simulink model "project2_animation"  (R2017a)
settings: Solver=FixedStepDiscrete  StartTime=0.0  StopTime=1000.0  FixedStep=0.1  RelTol=1e-3
undefined symbols (not defined in the file or in its folder): drawVehicle
libraries: simulink x6
settings Model: Creator=pizzaslayer  LastModifiedBy=pizzaslayer

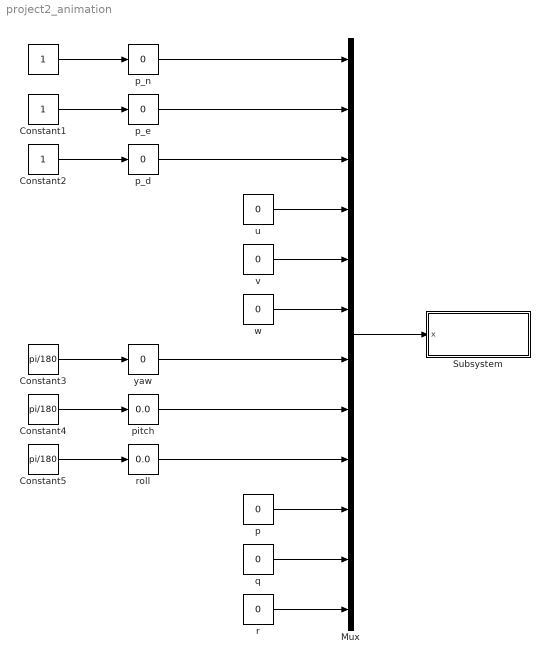
== system project2_animation ==
  " " : Constant
  Constant1 : Constant
  Constant2 : Constant
  Constant3 : Constant  Value=pi/180
  Constant4 : Constant  Value=pi/180
  Constant5 : Constant  Value=pi/180
  Mux : Mux  Inputs=12
  Subsystem : Subsystem
  p : Constant  Value=0
  p_d : simulink/Math Operations/Slider Gain  gain=0  low=-10  high=10
  p_e : simulink/Math Operations/Slider Gain  gain=0  low=-10  high=10
  p_n : simulink/Math Operations/Slider Gain  gain=0  low=-10  high=10
  pitch : simulink/Math Operations/Slider Gain  gain=0.0  low=-180  high=180
  q : Constant  Value=0
  r : Constant  Value=0
  roll : simulink/Math Operations/Slider Gain  gain=0.0  low=-180  high=180
  u : Constant  Value=0
  v : Constant  Value=0
  w : Constant  Value=0
  yaw : simulink/Math Operations/Slider Gain  gain=0  low=-180  high=180
  wires:
  p_n/1 -> Mux/1
  " "/1 -> p_n/1
  Constant3/1 -> yaw/1
  yaw/1 -> Mux/7
  pitch/1 -> Mux/8
  Constant4/1 -> pitch/1
  Constant5/1 -> roll/1
  roll/1 -> Mux/9
  p_e/1 -> Mux/2
  Constant1/1 -> p_e/1
  Constant2/1 -> p_d/1
  p_d/1 -> Mux/3
  p/1 -> Mux/10
  q/1 -> Mux/11
  r/1 -> Mux/12
  w/1 -> Mux/6
  v/1 -> Mux/5
  u/1 -> Mux/4
  Mux/1 -> Subsystem/1(x)

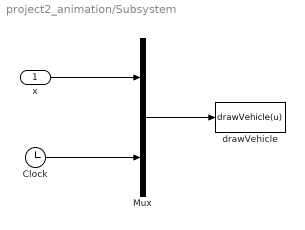
== system project2_animation/Subsystem ==
  x : Inport
  Clock : Clock
  Mux : Mux  Inputs=2
  drawVehicle : MATLABFcn  MATLABFcn=drawVehicle(u)  OutputDimensions=0
  wires:
  Clock/1 -> Mux/2
  x/1 -> Mux/1
  Mux/1 -> drawVehicle/1
